simulink model "serienschwingkreis"  (R2016b)
settings: Solver=VariableStepAuto  StartTime=0.0  StopTime=10.0  RelTol=1e-3
values from neighbouring files (symbols this model uses):
  C = 0.6    [automodell_param.m]    (also in serienschwingkreis_param.m = 0.005)
  L = 2    [serienschwingkreis_param.m]
  R = 5    [serienschwingkreis_param.m]
  Rkrit = 2*sqrt(L/C)    [serienschwingkreis_param.m]
settings Model: Creator=local  LastModifiedBy=local

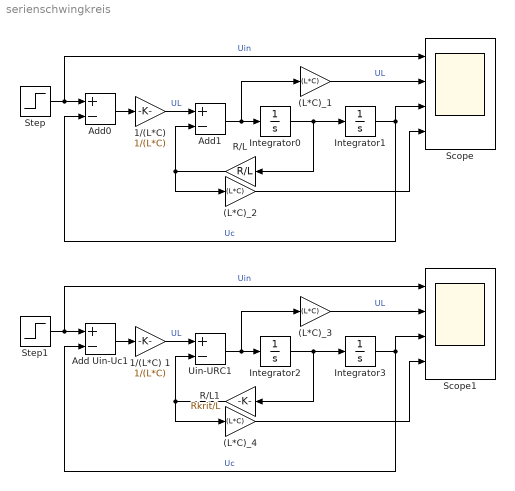
== system serienschwingkreis ==
  (L*C)_{1..4} (4 alike) : Gain  Gain=(L*C)
  "1/(L*C) " : Gain  Gain=1/(L*C)
  1/(L*C) 1 : Gain  Gain=1/(L*C)
  Add Uin-Uc1 : Sum  Inputs=+-
  Add0 : Sum  Inputs=+-
  Add1 : Sum  Inputs=+-
  Integrator{0..3} (4 alike) : Integrator
  R/L : Gain  Gain=R/L
  R/L1 : Gain  Gain=Rkrit/L
  Scope : Scope  NumInputPorts=4
  Scope1 : Scope  NumInputPorts=4
  Step : Step  After=10  SampleTime=0.00001
  Step1 : Step  After=10  SampleTime=0.00001
  Uin-URC1 : Sum  Inputs=+-
  wires:
  "1/(L*C) "/1 -> Add1/1  "UL"
  Step/1 -> Scope/1, Add0/1  "Uin"
  Add0/1 -> "1/(L*C) "/1
  Add1/1 -> (L*C)_1/1, Integrator0/1
  Integrator0/1 -> Integrator1/1, R/L/1
  R/L/1 -> (L*C)_2/1, Add1/2
  Integrator1/1 -> Scope/3, Add0/2  "Uc"
  (L*C)_1/1 -> Scope/2  "UL"
  (L*C)_2/1 -> Scope/4
  1/(L*C) 1/1 -> Uin-URC1/1  "UL"
  Step1/1 -> Scope1/1, Add Uin-Uc1/1  "Uin"
  Add Uin-Uc1/1 -> 1/(L*C) 1/1
  Uin-URC1/1 -> (L*C)_3/1, Integrator2/1
  Integrator2/1 -> Integrator3/1, R/L1/1
  R/L1/1 -> (L*C)_4/1, Uin-URC1/2
  Integrator3/1 -> Scope1/3, Add Uin-Uc1/2  "Uc"
  (L*C)_3/1 -> Scope1/2  "UL"
  (L*C)_4/1 -> Scope1/4
